simulink model "STC_Santhosh1"  (R2024b)
settings: Solver=VariableStepAuto  StartTime=0.0  StopTime=10  RelTol=1e-3
(part 2 of 2)

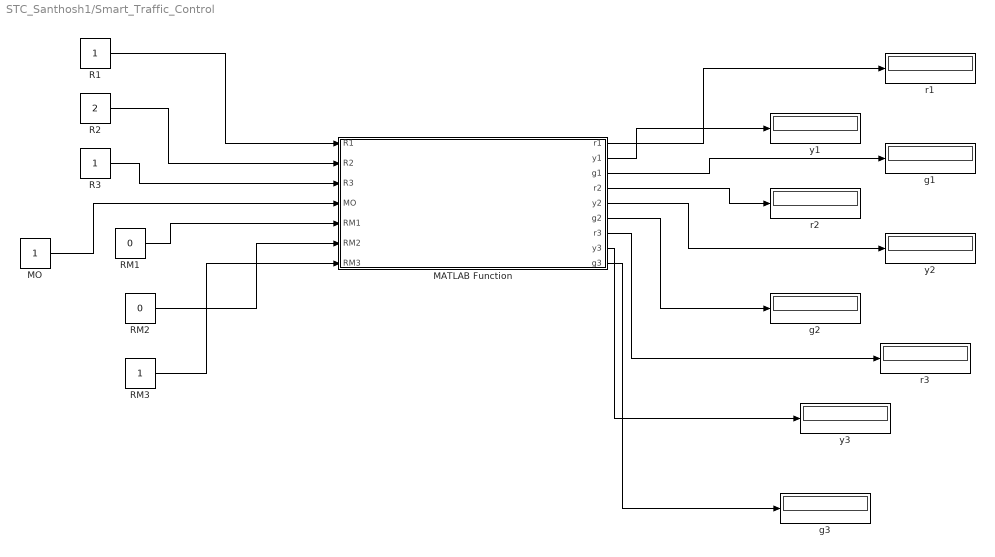
== system STC_Santhosh1/Smart_Traffic_Control ==
  MATLAB Function : MATLAB Function  TreatAsAtomicUnit=on
  MO : Constant
  R1 : Constant
  R2 : Constant  Value=2
  R3 : Constant
  RM1 : Constant  Value=0
  RM2 : Constant  Value=0
  RM3 : Constant
  g1 : Display
  g2 : Display
  g3 : Display
  r1 : Display
  r2 : Display
  r3 : Display
  y1 : Display
  y2 : Display
  y3 : Display
  wires:
  MATLAB Function/8(y3) -> y3/1
  RM3/1 -> MATLAB Function/7(RM3)
  MATLAB Function/7(r3) -> r3/1
  MATLAB Function/9(g3) -> g3/1
  MATLAB Function/4(r2) -> r2/1
  MATLAB Function/2(y1) -> y1/1
  MATLAB Function/5(y2) -> y2/1
  MATLAB Function/1(r1) -> r1/1
  MATLAB Function/3(g1) -> g1/1
  MATLAB Function/6(g2) -> g2/1
  RM2/1 -> MATLAB Function/6(RM2)
  R2/1 -> MATLAB Function/2(R2)
  R1/1 -> MATLAB Function/1(R1)
  RM1/1 -> MATLAB Function/5(RM1)
  MO/1 -> MATLAB Function/4(MO)
  R3/1 -> MATLAB Function/3(R3)

== matlab function STC_Santhosh1/Smart_Traffic_Control/MATLAB Function ==
  data: R1 input; r1 output; R2 input; R3 input; MO input; RM1 input; RM2 input; RM3 input; y1 output; g1 output; r2 output; y2 output; g2 output; r3 output; y3 output; g3 output
function [r1,y1,g1,r2,y2,g2,r3,y3,g3] = fcn(R1,R2,R3,MO,RM1,RM2,RM3)


r1 = 0; y1 = 0; g1 = 0;
r2 = 0; y2 = 0; g2 = 0;
r3 = 0; y3 = 0; g3 = 0;


if MO ==0    
   if R1 > R2 && R1 > R3
        r1 = 0; y1 = 0; g1 = 1;
        r2 = 1; y2 = 0; g2 = 0;
        r3 = 0; y3 = 1; g3 = 0;
    elseif R2 > R3 && R2>R1
        r1 = 0; y1 = 1; g1 = 0;
        r2 = 0; y2 = 0; g2 = 1;
        r3 = 1; y3 = 0; g3 = 0;
    elseif R3 > R1 && R3 > R2
        r1 = 1; y1 = 0; g1 = 0;
        r2 = 0; y2 = 1; g2 = 0;
        r3 = 0; y3 = 0; g3 = 1;
   end
elseif MO ==1
    if RM1 == 1
        r1 = 0; y1 = 0; g1 = 1;
        r2 = 1; y2 = 0; g2 = 0;
        r3 = 0; y3 = 1; g3 = 0;
    elseif RM2 == 1  
        r1 = 0; y1 = 1; g1 = 0;
        r2 = 0; y2 = 0; g2 = 1;
        r3 = 1; y3 = 0; g3 = 0;
    elseif RM3 == 1
        r1 = 1; y1 = 0; g1 = 0;
        r2 = 0; y2 = 1; g2 = 0;
        r3 = 0; y3 = 0; g3 = 1;
   
    end
end


end
